simulink model "ControlDC_Velocidad_RTWT_6221_2017b"  (R2017b)
settings: Solver=ode5  StartTime=0.0  StopTime=inf  FixedStep=T  RelTol=1e-3  EnableMultiTasking=on
undefined symbols (not defined in the file or in its folder): National_Instruments, PCI, T
libraries: sldrtlib x3, simulink x1, simulink_need_slupdate x1
settings Model: SimulationMode=external  Creator=Rafa  LastModifiedBy=EIB
settings DataIOCC: LimitDataPoints=on  SaveFormat=Array  SignalLoggingSaveFormat=ModelDataLogs
settings OptimizationCC: ExpressionDepthLimit=2147483647
settings DebuggingCC: UnderspecifiedInitializationDetection=Classic  MergeDetectMultiDrivingBlocksExec=none  SolverPrmCheckMsg=warning  FcnCallInpInsideContextMsg=warning  StateNameClashWarn=warning  SFUnexpectedBacktrackingDiag=warning  SFNoUnconditionalDefaultTransitionDiag=warning  SFExecutionAtInitializationDiag=none
settings ModelReferenceCC: PropagateSignalLabelsOutOfModel=off
settings RTWCC: SystemTargetFile=sldrt.tlc  TemplateMakefile=sldrt.tmf  Description=Simulink Desktop Real-Time  RTWCompilerOptimization=on
settings CodeAppCC: MaxIdLength=95  StateflowObjectComments=on
settings SimulinkDesktopRealTimeCC: TargetPreCompLibLocation=C:\MATLAB\R2017b\toolbox\sldrt\lib\win64  TargetLangStandard=C89/C90 (ANSI)  SupportVariableSizeSignals=off
settings ConfigComp: CovMetricSettings=dw  CovHtmlReporting=on  CovSaveCumulativeToWorkspaceVar=on  CovSaveSingleToWorkspaceVar=on  CovExternalEMLEnable=off

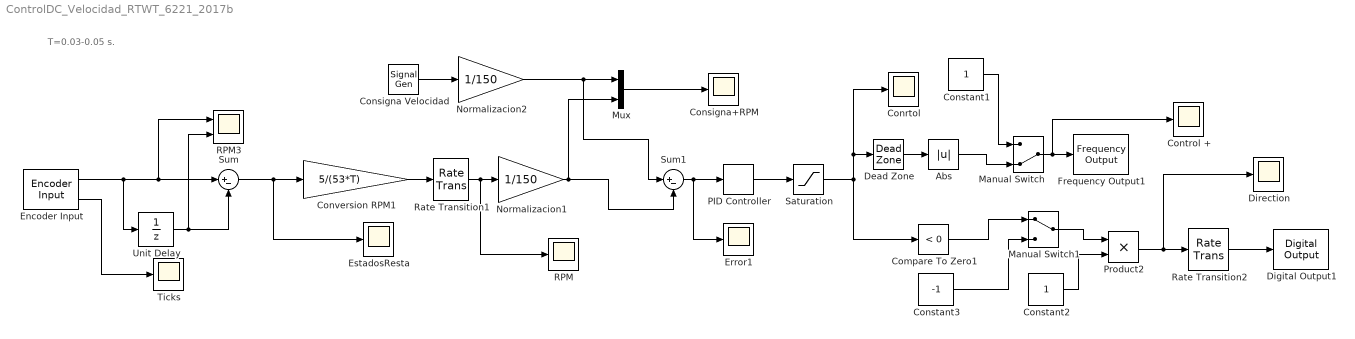
== system ControlDC_Velocidad_RTWT_6221_2017b ==
  note: T=0.03-0.05 s.
  Abs : Abs
  Compare To Zero1 : simulink/Logic and Bit Operations/Compare To Zero  relop=<  OutDataTypeStr=uint8
  Conrtol : Scope
  Consigna Velocidad : SignalGenerator  WaveForm=square  Amplitude=140  Frequency=0.3
  Consigna+RPM : Scope
  Constant1 : Constant
  Constant2 : Constant
  Constant3 : Constant  Value=-1
  Control + : Scope
  Conversion RPM1 : Gain  Gain=5/(53*T)
  Dead Zone : DeadZone  LowerValue=-0.1  UpperValue=0.1  SaturateOnIntegerOverflow=on
  Digital Output1 : sldrtlib/Digital Output  SampleTime=T  MaxMissedTicks=10  ShowMissedTicks=off  YieldWhenWaiting=off  DrvName=National_Instruments/PCI-6221  DrvAddress=4294967295  DrvOptions=[1 1 20480 3 1]  Channels=1  BitMode=1  InitialValue=0  FinalValue=0
      settings: AttributesFormatString=National Instruments\nPCI-6221 [auto]  SourceProductName=Simulink Desktop Real-Time  SourceProductBaseCode=WT
  Direction : Scope
  Encoder Input : sldrtlib/Encoder Input  SampleTime=T  MaxMissedTicks=10  ShowMissedTicks=on  YieldWhenWaiting=off  DrvName=National_Instruments/PCI-6221  DrvAddress=4294967295  DrvOptions=[1 1 20480 3 2]  Channels=2  QuadMode=3  IndexPulse=1  InputFilter=Inf  DataType=1
      settings: AttributesFormatString=National Instruments\nPCI-6221 [auto]  SourceProductName=Simulink Desktop Real-Time
  Error1 : Scope
  EstadosResta : Scope
  Frequency Output1 : sldrtlib/Frequency Output  SampleTime=-1  MaxMissedTicks=10  ShowMissedTicks=off  YieldWhenWaiting=off  DrvName=National_Instruments/PCI-6221  DrvAddress=4294967295  DrvOptions=[1 1 20480 3 1]  Channels=1  FrequencySource=1  Frequency=100  FrequencyFinalValue=[]  DutySource=2  Duty=0  DutyFinalValue=0
      settings: AttributesFormatString=National Instruments\nPCI-6221 [auto]  SourceProductName=Simulink Desktop Real-Time  SourceProductBaseCode=WT
  Manual Switch : ManualSwitch  CurrentSetting=0
  Manual Switch1 : ManualSwitch
  Mux : Mux  Inputs=2
  Normalizacion1 : Gain  Gain=1/150
  Normalizacion2 : Gain  Gain=1/150
  PID Controller : simulink_need_slupdate/PID Controller  P=0.5  I=5  D=0
      settings: SourceProductName=Simulink
  Product2 : Product  RndMeth=Zero
  RPM : Scope
  RPM3 : Scope  NumInputPorts=2
  Rate Transition1 : RateTransition  OutPortSampleTime=T
  Rate Transition2 : RateTransition  OutPortSampleTime=T
  Saturation : Saturate  UpperLimit=1  LowerLimit=-1
  Sum : Sum  Inputs=|+-
  Sum1 : Sum  Inputs=|+-
  Ticks : Scope
  Unit Delay : UnitDelay  SampleTime=T
  wires:
  Product2/1 -> Rate Transition2/1, Direction/1
  Constant2/1 -> Product2/2
  Saturation/1 -> Conrtol/1, Dead Zone/1, Compare To Zero1/1
  Rate Transition2/1 -> Digital Output1/1
  Consigna Velocidad/1 -> Normalizacion2/1
  Sum1/1 -> PID Controller/1, Error1/1
  Normalizacion2/1 -> Mux/1, Sum1/1
  PID Controller/1 -> Saturation/1
  Mux/1 -> Consigna+RPM/1
  Encoder Input/1 -> RPM3/1, Sum/1, Unit Delay/1
  Unit Delay/1 -> RPM3/2, Sum/2
  Sum/1 -> Conversion RPM1/1, EstadosResta/1
  Conversion RPM1/1 -> Rate Transition1/1
  Normalizacion1/1 -> Mux/2, Sum1/2
  Dead Zone/1 -> Abs/1
  Rate Transition1/1 -> RPM/1, Normalizacion1/1
  Manual Switch/1 -> Control +/1, Frequency Output1/1
  Abs/1 -> Manual Switch/2
  Manual Switch1/1 -> Product2/1
  Compare To Zero1/1 -> Manual Switch1/1
  Constant1/1 -> Manual Switch/1
  Encoder Input/2 -> Ticks/1
  Constant3/1 -> Manual Switch1/2
